simulink model "Part3"  (R2024a)
settings: Solver=VariableStepAuto  StartTime=0.0  StopTime=20  RelTol=1e-3
undefined symbols (not defined in the file or in its folder): magnitude
settings Model: Creator=katutu  LastModifiedBy=katutu

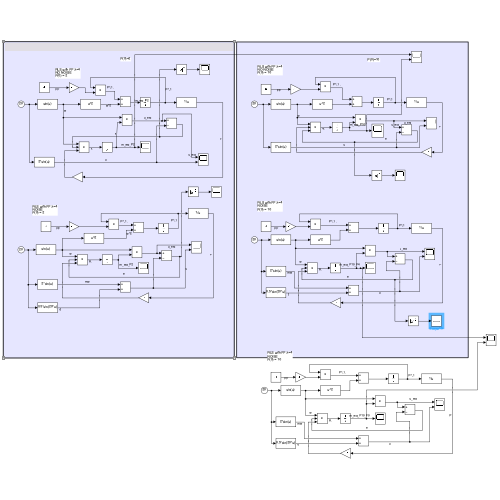
[thumbnail: Simulink's stored preview of the top-level diagram]
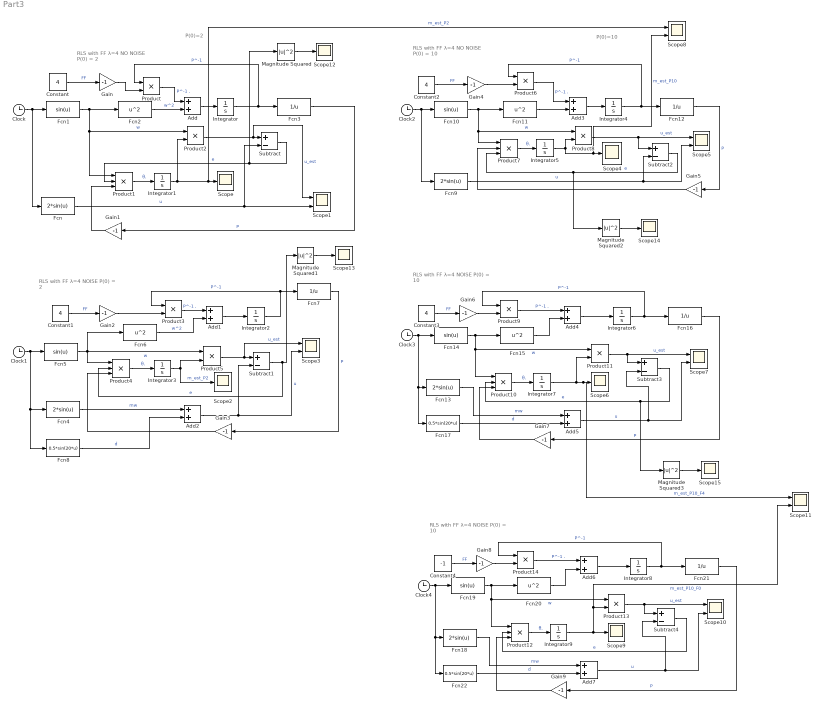
== system Part3 ==
  note: P(0)=10
  note: P(0)=2
  note: RLS with FF λ=4
      | NO NOISE
      | P(0) = 2
  note: RLS with FF λ=4
      | NOISE
      | P(0) = 2
  note: RLS with FF λ=4
      | NOISE
      | P(0) = 10
  note: RLS with FF λ=4
      | NO NOISE
      | P(0) = 10
  note: RLS with FF λ=4
      | NOISE
      | P(0) = 10
  Add{,1..7} (8 alike) : Sum
  Clock{,1..4} (5 alike) : Clock
  Constant{,1..3} (4 alike) : Constant  Value=4
  Constant4 : Constant  Value=-1
  Fcn{,4,9,13,18} (5 alike) : Fcn  Expr=2*sin(u)
  Fcn{1,5,10,14,19} (5 alike) : Fcn  Expr=sin(u)
  Fcn{2,6,11,15,20} (5 alike) : Fcn  Expr=u^2
  Fcn{3,7,12,16,21} (5 alike) : Fcn  Expr=1/u
  Fcn17 : Fcn  Expr=0.5*sin(20*u)
  Fcn22 : Fcn  Expr=0.5*sin(20*u)
  Fcn8 : Fcn  Expr=0.5*sin(20*u)
  Gain{,1..9} (10 alike) : Gain  Gain=-1
  Integrator{,1..3,5,7,9} (7 alike) : Integrator  InitialCondition=0.5
  Integrator4 : Integrator  InitialCondition=0.1
  Integrator6 : Integrator  InitialCondition=0.1
  Integrator8 : Integrator  InitialCondition=0.1
  Magnitude Squared{,1..3} (4 alike) : Math  Operator=magnitude^2
  Product{,2..3,5..6,8..9,11,13..14} (10 alike) : Product
  Product{1,4,7,10,12} (5 alike) : Product  Inputs=3
  Scope{,2,4,6,9,12..15} (9 alike) : Scope
  Scope{1,3,5,7..8,10..11} (7 alike) : Scope  NumInputPorts=2
  Subtract{,1..4} (5 alike) : Sum  Inputs=+-
  wires:
  Subtract/1 -> Magnitude Squared/1, Product1/2  "e"
  Fcn3/1 -> Gain1/1  "P"
  Product/1 -> Add/1  "P^-1 ."
  Product1/1 -> Integrator1/1  "θ."
  Gain/1 -> Product/2
  Product2/1 -> Scope1/1, Subtract/1  "u_est"
  Fcn/1 -> Scope1/2, Subtract/2  "u"
  Integrator/1 -> Product/1, Fcn3/1  "P^-1"
  Add/1 -> Integrator/1
  Fcn2/1 -> Add/2  "w^2"
  Fcn1/1 -> Fcn2/1, Product1/1, Product2/1  "w"
  Constant/1 -> Gain/1  "FF"
  Integrator1/1 -> Scope8/1, Scope/1, Product2/2  "m_est_P2"
  Clock/1 -> Fcn1/1, Fcn/1
  Gain1/1 -> Product1/3
  Integrator2/1 -> Product3/1, Fcn7/1  "P^-1"
  Add1/1 -> Integrator2/1
  Product4/1 -> Integrator3/1  "θ."
  Subtract1/1 -> Magnitude Squared1/1, Product4/2  "e"
  Fcn5/1 -> Product4/1, Product5/1, Fcn6/1  "w"
  Product3/1 -> Add1/1  "P^-1 ."
  Product5/1 -> Scope3/1, Subtract1/1  "u_est"
  Gain2/1 -> Product3/2
  Fcn7/1 -> Gain3/1  "P"
  Constant1/1 -> Gain2/1  "FF"
  Integrator3/1 -> Scope2/1, Product5/2  "m_est_P2"
  Clock1/1 -> Fcn8/1, Fcn4/1, Fcn5/1
  Gain3/1 -> Product4/3
  Fcn6/1 -> Add1/2  "w^2"
  Fcn4/1 -> Add2/1  "mw"
  Add2/1 -> Scope3/2, Subtract1/2  "u"
  Fcn8/1 -> Add2/2  "d"
  Integrator7/1 -> Scope11/1, Scope6/1, Product11/2  "m_est_P10_F4"
  Add3/1 -> Integrator4/1
  Clock2/1 -> Fcn10/1, Fcn9/1
  Gain5/1 -> Product7/2
  Fcn16/1 -> Gain7/1  "P"
  Clock3/1 -> Fcn17/1, Fcn13/1, Fcn14/1
  Integrator6/1 -> Fcn16/1, Product9/1  "P^-1"
  Product9/1 -> Add4/1  "P^-1 ."
  Fcn15/1 -> Add4/2
  Integrator5/1 -> Scope8/2, Scope4/1, Product8/2  "m_est_P10"
  Gain7/1 -> Product10/3
  Constant3/1 -> Gain6/1  "FF"
  Fcn12/1 -> Gain5/1  "P"
  Add4/1 -> Integrator6/1
  Product6/1 -> Add3/1  "P^-1 ."
  Fcn14/1 -> Product10/1, Product11/1, Fcn15/1  "w"
  Subtract3/1 -> Magnitude Squared3/1, Product10/2  "e"
  Gain6/1 -> Product9/2
  Product11/1 -> Scope7/1, Subtract3/1  "u_est"
  Product8/1 -> Scope5/1, Subtract2/1  "u_est"
  Add5/1 -> Scope7/2, Subtract3/2  "u"
  Product7/1 -> Integrator5/1  "θ."
  Product10/1 -> Integrator7/1  "θ."
  Gain4/1 -> Product6/2
  Subtract2/1 -> Magnitude Squared2/1, Product7/3  "e"
  Integrator4/1 -> Fcn12/1, Product6/1  "P^-1"
  Constant2/1 -> Gain4/1  "FF"
  Fcn10/1 -> Fcn11/1, Product7/1, Product8/1  "w"
  Fcn9/1 -> Scope5/2, Subtract2/2  "u"
  Fcn11/1 -> Add3/2
  Fcn13/1 -> Add5/1  "mw"
  Fcn17/1 -> Add5/2  "d"
  Fcn18/1 -> Add7/1  "mw"
  Fcn19/1 -> Product12/1, Product13/1, Fcn20/1  "w"
  Constant4/1 -> Gain8/1  "FF"
  Product14/1 -> Add6/1  "P^-1 ."
  Product12/1 -> Integrator9/1  "θ."
  Integrator9/1 -> Scope9/1, Scope11/2, Product13/2  "m_est_P10_F0"
  Product13/1 -> Scope10/1, Subtract4/1  "u_est"
  Subtract4/1 -> Product12/2  "e"
  Fcn21/1 -> Gain9/1  "P"
  Gain9/1 -> Product12/3
  Clock4/1 -> Fcn22/1, Fcn18/1, Fcn19/1
  Fcn20/1 -> Add6/2
  Add7/1 -> Scope10/2, Subtract4/2  "u"
  Fcn22/1 -> Add7/2  "d"
  Add6/1 -> Integrator8/1
  Integrator8/1 -> Fcn21/1, Product14/1  "P^-1"
  Gain8/1 -> Product14/2
  Magnitude Squared/1 -> Scope12/1
  Magnitude Squared1/1 -> Scope13/1
  Magnitude Squared2/1 -> Scope14/1
  Magnitude Squared3/1 -> Scope15/1
